simulink subsystem "angleOffsetsCADtoSimscape"  (R2024a)
settings: Solver=VariableStepAuto  StartTime=0.0  StopTime=10.0  RelTol=1e-3
libraries: simulink_extras x3
settings Model: Creator=ckammer  LastModifiedBy=ckammer

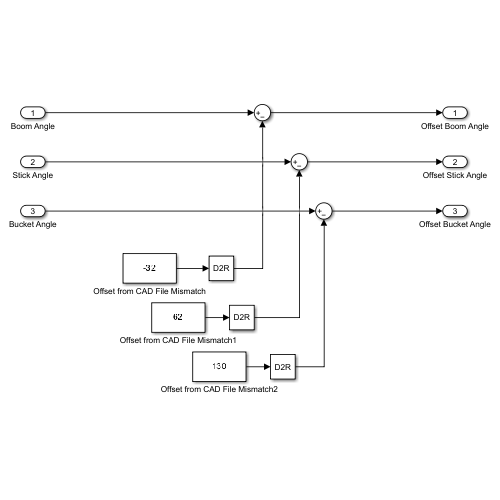
[thumbnail: Simulink's stored preview of the top-level diagram]
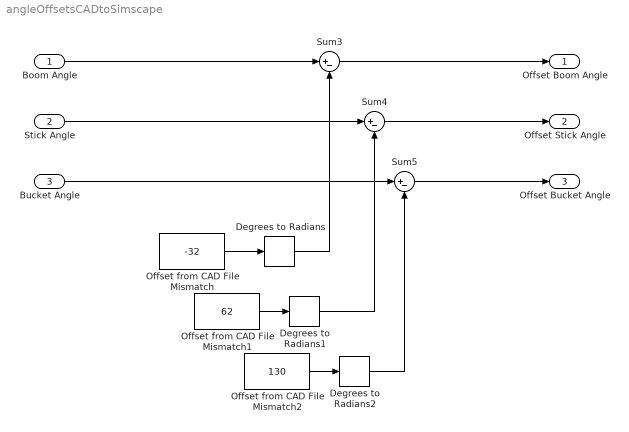
== system angleOffsetsCADtoSimscape ==
  Boom Angle : Inport
  Stick Angle : Inport  Port=2
  Bucket Angle : Inport  Port=3
  Degrees to Radians : simulink_extras/Transformations/Degrees to Radians
  Degrees to Radians1 : simulink_extras/Transformations/Degrees to Radians
  Degrees to Radians2 : simulink_extras/Transformations/Degrees to Radians
  Offset from CAD File Mismatch : Constant  Value=-32
  Offset from CAD File Mismatch1 : Constant  Value=62
  Offset from CAD File Mismatch2 : Constant  Value=130
  Sum3 : Sum  Inputs=|+-
  Sum4 : Sum  Inputs=|+-
  Sum5 : Sum  Inputs=|+-
  Offset Boom Angle : Outport
  Offset Stick Angle : Outport  Port=2
  Offset Bucket Angle : Outport  Port=3
  wires:
  Stick Angle/1 -> Sum4/1
  Bucket Angle/1 -> Sum5/1
  Degrees to Radians/1 -> Sum3/2
  Offset from CAD File Mismatch2/1 -> Degrees to Radians2/1
  Offset from CAD File Mismatch/1 -> Degrees to Radians/1
  Offset from CAD File Mismatch1/1 -> Degrees to Radians1/1
  Sum4/1 -> Offset Stick Angle/1
  Degrees to Radians2/1 -> Sum5/2
  Sum3/1 -> Offset Boom Angle/1
  Boom Angle/1 -> Sum3/1
  Degrees to Radians1/1 -> Sum4/2
  Sum5/1 -> Offset Bucket Angle/1
